simulink model "q4"  (R2022a)
settings: Solver=VariableStepAuto  StartTime=0.0  StopTime=10.0  RelTol=1e-3
undefined symbols (not defined in the file): designMultirateFIR
libraries: dspmlti4 x5
settings Model: Creator=Ariike.ir  LastModifiedBy=Ariike.ir

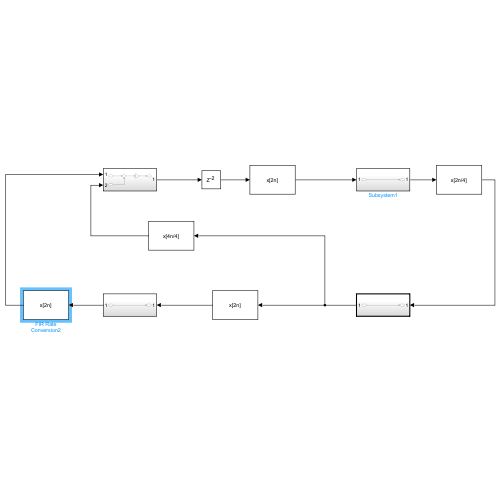
[thumbnail: Simulink's stored preview of the top-level diagram]
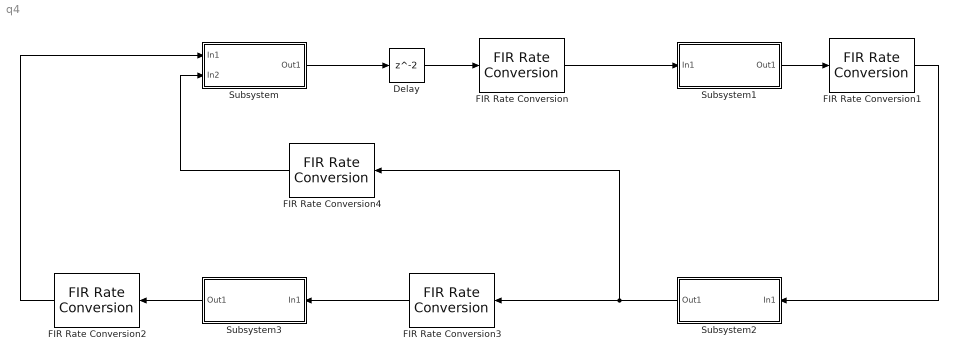
== system q4 ==
  Delay : Delay
  FIR Rate Conversion : dspmlti4/FIR Rate Conversion  FilterSource=Auto  L=1  h=designMultirateFIR(3,2)  M=2  FilterObject=FRC  rateMode=Enforce single-rate processing  roundingMode=Floor  overflowMode=off  firstCoeffDataTypeStr=Inherit: Same word length as input  firstCoeffMin=[]  firstCoeffMax=[]  firstCoeffLastDataTypeStr=Inherit: Same word length as input  outputDataTypeStr=Inherit: Same as accumulator  outputMin=[]  outputMax=[]  outputLastDataTypeStr=Inherit: Same as accumulator
      settings: SourceProductBaseCode=DS
  FIR Rate Conversion1 : dspmlti4/FIR Rate Conversion  FilterSource=Auto  L=4  h=designMultirateFIR(3,2)  M=2  FilterObject=FRC  rateMode=Enforce single-rate processing  roundingMode=Floor  overflowMode=off  firstCoeffDataTypeStr=Inherit: Same word length as input  firstCoeffMin=[]  firstCoeffMax=[]  firstCoeffLastDataTypeStr=Inherit: Same word length as input  outputDataTypeStr=Inherit: Same as accumulator  outputMin=[]  outputMax=[]  outputLastDataTypeStr=Inherit: Same as accumulator
      settings: SourceProductBaseCode=DS
  FIR Rate Conversion2 : dspmlti4/FIR Rate Conversion  FilterSource=Auto  L=1  h=designMultirateFIR(3,2)  M=2  FilterObject=FRC  rateMode=Enforce single-rate processing  roundingMode=Floor  overflowMode=off  firstCoeffDataTypeStr=Inherit: Same word length as input  firstCoeffMin=[]  firstCoeffMax=[]  firstCoeffLastDataTypeStr=Inherit: Same word length as input  outputDataTypeStr=Inherit: Same as accumulator  outputMin=[]  outputMax=[]  outputLastDataTypeStr=Inherit: Same as accumulator
      settings: SourceProductBaseCode=DS
  FIR Rate Conversion3 : dspmlti4/FIR Rate Conversion  FilterSource=Auto  L=1  h=designMultirateFIR(3,2)  M=2  FilterObject=FRC  rateMode=Enforce single-rate processing  roundingMode=Floor  overflowMode=off  firstCoeffDataTypeStr=Inherit: Same word length as input  firstCoeffMin=[]  firstCoeffMax=[]  firstCoeffLastDataTypeStr=Inherit: Same word length as input  outputDataTypeStr=Inherit: Same as accumulator  outputMin=[]  outputMax=[]  outputLastDataTypeStr=Inherit: Same as accumulator
      settings: SourceProductBaseCode=DS
  FIR Rate Conversion4 : dspmlti4/FIR Rate Conversion  FilterSource=Auto  L=4  h=designMultirateFIR(3,2)  M=4  FilterObject=FRC  rateMode=Enforce single-rate processing  roundingMode=Floor  overflowMode=off  firstCoeffDataTypeStr=Inherit: Same word length as input  firstCoeffMin=[]  firstCoeffMax=[]  firstCoeffLastDataTypeStr=Inherit: Same word length as input  outputDataTypeStr=Inherit: Same as accumulator  outputMin=[]  outputMax=[]  outputLastDataTypeStr=Inherit: Same as accumulator
      settings: SourceProductBaseCode=DS
  Subsystem : Subsystem
  Subsystem1 : Subsystem
  Subsystem2 : Subsystem
  Subsystem3 : Subsystem
  wires:
  Subsystem/1(Out1) -> Delay/1
  Delay/1 -> FIR Rate Conversion/1
  FIR Rate Conversion/1 -> Subsystem1/1(In1)
  FIR Rate Conversion1/1 -> Subsystem2/1(In1)
  FIR Rate Conversion2/1 -> Subsystem/1(In1)
  FIR Rate Conversion3/1 -> Subsystem3/1(In1)
  FIR Rate Conversion4/1 -> Subsystem/2(In2)
  Subsystem1/1(Out1) -> FIR Rate Conversion1/1
  Subsystem3/1(Out1) -> FIR Rate Conversion2/1
  Subsystem2/1(Out1) -> FIR Rate Conversion4/1, FIR Rate Conversion3/1

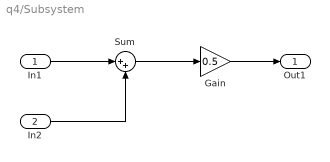
== system q4/Subsystem ==
  In1 : Inport
  In2 : Inport  Port=2
  Gain : Gain  Gain=0.5
  Sum : Sum  Inputs=|++
  Out1 : Outport
  wires:
  In2/1 -> Sum/2
  Sum/1 -> Gain/1
  In1/1 -> Sum/1
  Gain/1 -> Out1/1

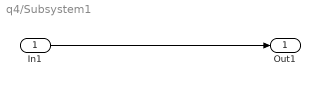
== system q4/Subsystem1 ==
  In1 : Inport
  Out1 : Outport
  wires:
  In1/1 -> Out1/1

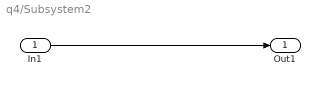
== system q4/Subsystem2 ==
  In1 : Inport
  Out1 : Outport
  wires:
  In1/1 -> Out1/1

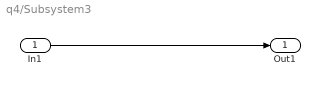
== system q4/Subsystem3 ==
  In1 : Inport
  Out1 : Outport
  wires:
  In1/1 -> Out1/1
